simulink model "openMHA_test_db_lookup"  (R2020a)
settings: Solver=VariableStepAuto  StartTime=0.0  StopTime=stop_time  RelTol=1e-3
InitFcn:
  | test_db_lookup_init
StopFcn:
  | test_db_lookup_stop
values from neighbouring files (symbols this model uses):
  xIn = [4.65661287308e-10 5.23868948221e-10 5.82076609135e-10 6.40284270048e-10 6.98491930962e-10 7.56699591875e-10 8.14907252789e-10 8.73114913702e-10 9.31322574615e-10 1.04773789644e-09 1.16415321827e-09 1.2805685401e-09 ... (256 elements, 1x256)]    [openMHA_test_db_lookup_gain_Programmable Look-Up Table_init.mat]    (also in openMHA_test_db_lookup_gain_Programmable Lookup Table dB_init.mat = [4.65661287308e-10 4.72937244922e-10 4.80213202536e-10 4.874)
libraries: FPGA_Open_Speech_Tools x1, dspsrcs4 x1
settings Model: PacingRate=35  Creator=t96f346  LastModifiedBy=t96f346

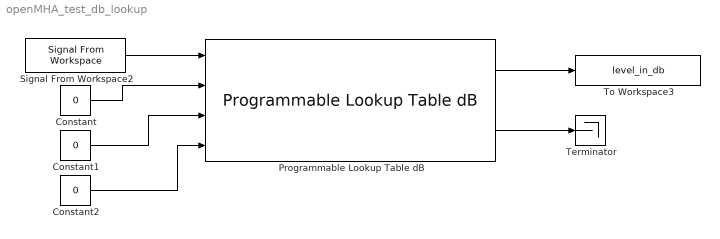
== system openMHA_test_db_lookup ==
  Constant : Constant  Value=0  SampleTime=-1
  Constant1 : Constant  Value=0  SampleTime=-1
  Constant2 : Constant  Value=0  OutDataTypeStr=boolean  SampleTime=-1
  Programmable Lookup Table dB : FPGA_Open_Speech_Tools/Programmable Lookup Table dB  tableFnParam=10.*log10(2500000000.*xIn)  SAVE_TABLE=off  maxInput=1  floorParam=2^-31  errorParam=1  ERR_DIAG=on  PLOT_TABLE=off  nBitsParam=5  mBitsParam=4  IGOTTHIS=off  W_bits=40  F_bits=37  tableInit=0  binaryOffset=0
      settings: SourceProductName=FPGA Open Speech Tools
  Signal From Workspace2 : dspsrcs4/Signal From Workspace  X=level_in  Ts=1  nsamps=1  OutputAfterFinalValue=Setting to zero  ignoreOrWarnInputAndFrameLengths=off  OutputFrames=off
  Terminator : Terminator
  To Workspace3 : ToWorkspace  VariableName=level_in_db  SampleTime=-1
      settings: Save2DSignal=2-D array (concatenate along first dimension)
  wires:
  Signal From Workspace2/1 -> Programmable Lookup Table dB/1
  Programmable Lookup Table dB/1 -> To Workspace3/1
  Programmable Lookup Table dB/2 -> Terminator/1
  Constant/1 -> Programmable Lookup Table dB/2
  Constant1/1 -> Programmable Lookup Table dB/3
  Constant2/1 -> Programmable Lookup Table dB/4
